simulink model "aes_impl_decrypt_smc"  (R2015b)
settings: Solver=FixedStepDiscrete  SolverMode=SingleTasking  StartTime=0.0  StopTime=1000e-6  RelTol=1e-3
undefined symbols (not defined in the file): a, b, input_sample_rate
libraries: shlslibv1 x3018
(part 11 of 20)

== system aes_impl_decrypt_smc/Round12/Subsystem8/Subsystem5/Mixcolumn1 ==
  In1 : Inport
  In2 : Inport  Port=2
  In3 : Inport  Port=3
  In4 : Inport  Port=4
  Binary Logic : shlslibv1/Math Functions/Binary Logic  syn_binlog_exp=a^b  synBlockType=primitive  synLatency=0  synBlockId=13
  Binary Logic1 : shlslibv1/Math Functions/Binary Logic  syn_binlog_exp=a^b  synBlockType=primitive  synLatency=0  synBlockId=13
  Binary Logic2 : shlslibv1/Math Functions/Binary Logic  syn_binlog_exp=a^b  synBlockType=primitive  synLatency=0  synBlockId=13
  Display5 : Display
      settings: Format=hex (Stored Integer)
  Port Out : shlslibv1/Ports & Subsystems/Port Out  syn_capture=on  syn_register=on  synBlockType=port  synLatency=1  synBlockId=1
  multiplier1 : shlslibv1/Memories/ROM  syn_rom_vec=mul11  syn_rom_auto_wl=on  syn_out_wl=8  syn_out_fl=0  syn_out_dt=unsigned  syn_out_sat=on  syn_out_rnd=on  syn_en_port=off  synBlockType=primitive  synLatency=1  synBlockId=62  syn_dual_port=off
  multiplier2 : shlslibv1/Memories/ROM  syn_rom_vec=mul9  syn_rom_auto_wl=on  syn_out_wl=8  syn_out_fl=0  syn_out_dt=unsigned  syn_out_sat=on  syn_out_rnd=on  syn_en_port=off  synBlockType=primitive  synLatency=1  synBlockId=62  syn_dual_port=off
  multiplier3 : shlslibv1/Memories/ROM  syn_rom_vec=mul14  syn_rom_auto_wl=on  syn_out_wl=8  syn_out_fl=0  syn_out_dt=unsigned  syn_out_sat=on  syn_out_rnd=on  syn_en_port=off  synBlockType=primitive  synLatency=1  synBlockId=62  syn_dual_port=off
  multiplier4 : shlslibv1/Memories/ROM  syn_rom_vec=mul13  syn_rom_auto_wl=on  syn_out_wl=8  syn_out_fl=0  syn_out_dt=unsigned  syn_out_sat=on  syn_out_rnd=on  syn_en_port=off  synBlockType=primitive  synLatency=1  synBlockId=62  syn_dual_port=off
  Out1 : Outport
  wires:
  multiplier3/1 -> Binary Logic/2
  In2/1 -> multiplier3/1
  multiplier2/1 -> Binary Logic/1
  Binary Logic2/1 -> Port Out/1, Out1/1
  In1/1 -> multiplier2/1
  Port Out/1 -> Display5/1
  Binary Logic/1 -> Binary Logic2/1
  Binary Logic1/1 -> Binary Logic2/2
  multiplier1/1 -> Binary Logic1/1
  In3/1 -> multiplier1/1
  multiplier4/1 -> Binary Logic1/2
  In4/1 -> multiplier4/1

== system aes_impl_decrypt_smc/Round12/Subsystem8/Subsystem5/Mixcolumn2 ==
  In1 : Inport
  In2 : Inport  Port=2
  In3 : Inport  Port=3
  In4 : Inport  Port=4
  Binary Logic : shlslibv1/Math Functions/Binary Logic  syn_binlog_exp=a^b  synBlockType=primitive  synLatency=0  synBlockId=13
  Binary Logic1 : shlslibv1/Math Functions/Binary Logic  syn_binlog_exp=a^b  synBlockType=primitive  synLatency=0  synBlockId=13
  Binary Logic2 : shlslibv1/Math Functions/Binary Logic  syn_binlog_exp=a^b  synBlockType=primitive  synLatency=0  synBlockId=13
  Display5 : Display
      settings: Format=hex (Stored Integer)
  Port Out : shlslibv1/Ports & Subsystems/Port Out  syn_capture=on  syn_register=on  synBlockType=port  synLatency=1  synBlockId=1
  multiplier1 : shlslibv1/Memories/ROM  syn_rom_vec=mul14  syn_rom_auto_wl=on  syn_out_wl=8  syn_out_fl=0  syn_out_dt=unsigned  syn_out_sat=on  syn_out_rnd=on  syn_en_port=off  synBlockType=primitive  synLatency=1  synBlockId=62  syn_dual_port=off
  multiplier2 : shlslibv1/Memories/ROM  syn_rom_vec=mul13  syn_rom_auto_wl=on  syn_out_wl=8  syn_out_fl=0  syn_out_dt=unsigned  syn_out_sat=on  syn_out_rnd=on  syn_en_port=off  synBlockType=primitive  synLatency=1  synBlockId=62  syn_dual_port=off
  multiplier3 : shlslibv1/Memories/ROM  syn_rom_vec=mul9  syn_rom_auto_wl=on  syn_out_wl=8  syn_out_fl=0  syn_out_dt=unsigned  syn_out_sat=on  syn_out_rnd=on  syn_en_port=off  synBlockType=primitive  synLatency=1  synBlockId=62  syn_dual_port=off
  multiplier4 : shlslibv1/Memories/ROM  syn_rom_vec=mul11  syn_rom_auto_wl=on  syn_out_wl=8  syn_out_fl=0  syn_out_dt=unsigned  syn_out_sat=on  syn_out_rnd=on  syn_en_port=off  synBlockType=primitive  synLatency=1  synBlockId=62  syn_dual_port=off
  Out1 : Outport
  wires:
  multiplier3/1 -> Binary Logic/2
  In2/1 -> multiplier3/1
  multiplier2/1 -> Binary Logic/1
  Binary Logic2/1 -> Port Out/1, Out1/1
  In1/1 -> multiplier2/1
  Port Out/1 -> Display5/1
  Binary Logic/1 -> Binary Logic2/1
  Binary Logic1/1 -> Binary Logic2/2
  multiplier1/1 -> Binary Logic1/1
  In3/1 -> multiplier1/1
  multiplier4/1 -> Binary Logic1/2
  In4/1 -> multiplier4/1

== system aes_impl_decrypt_smc/Round12/Subsystem8/Subsystem5/Mixcolumn3 ==
  In1 : Inport
  In2 : Inport  Port=2
  In3 : Inport  Port=3
  In4 : Inport  Port=4
  Binary Logic : shlslibv1/Math Functions/Binary Logic  syn_binlog_exp=a^b  synBlockType=primitive  synLatency=0  synBlockId=13
  Binary Logic1 : shlslibv1/Math Functions/Binary Logic  syn_binlog_exp=a^b  synBlockType=primitive  synLatency=0  synBlockId=13
  Binary Logic2 : shlslibv1/Math Functions/Binary Logic  syn_binlog_exp=a^b  synBlockType=primitive  synLatency=0  synBlockId=13
  Display5 : Display
      settings: Format=hex (Stored Integer)
  Port Out : shlslibv1/Ports & Subsystems/Port Out  syn_capture=on  syn_register=on  synBlockType=port  synLatency=1  synBlockId=1
  multiplier1 : shlslibv1/Memories/ROM  syn_rom_vec=mul9  syn_rom_auto_wl=on  syn_out_wl=8  syn_out_fl=0  syn_out_dt=unsigned  syn_out_sat=on  syn_out_rnd=on  syn_en_port=off  synBlockType=primitive  synLatency=1  synBlockId=62  syn_dual_port=off
  multiplier2 : shlslibv1/Memories/ROM  syn_rom_vec=mul11  syn_rom_auto_wl=on  syn_out_wl=8  syn_out_fl=0  syn_out_dt=unsigned  syn_out_sat=on  syn_out_rnd=on  syn_en_port=off  synBlockType=primitive  synLatency=1  synBlockId=62  syn_dual_port=off
  multiplier3 : shlslibv1/Memories/ROM  syn_rom_vec=mul13  syn_rom_auto_wl=on  syn_out_wl=8  syn_out_fl=0  syn_out_dt=unsigned  syn_out_sat=on  syn_out_rnd=on  syn_en_port=off  synBlockType=primitive  synLatency=1  synBlockId=62  syn_dual_port=off
  multiplier4 : shlslibv1/Memories/ROM  syn_rom_vec=mul14  syn_rom_auto_wl=on  syn_out_wl=8  syn_out_fl=0  syn_out_dt=unsigned  syn_out_sat=on  syn_out_rnd=on  syn_en_port=off  synBlockType=primitive  synLatency=1  synBlockId=62  syn_dual_port=off
  Out1 : Outport
  wires:
  multiplier3/1 -> Binary Logic/2
  In2/1 -> multiplier3/1
  multiplier2/1 -> Binary Logic/1
  Binary Logic2/1 -> Port Out/1, Out1/1
  In1/1 -> multiplier2/1
  Port Out/1 -> Display5/1
  Binary Logic/1 -> Binary Logic2/1
  Binary Logic1/1 -> Binary Logic2/2
  multiplier1/1 -> Binary Logic1/1
  In3/1 -> multiplier1/1
  multiplier4/1 -> Binary Logic1/2
  In4/1 -> multiplier4/1

== system aes_impl_decrypt_smc/Round12/Subsystem8/Subsystem6/Mixcolumn ==
  In1 : Inport
  In2 : Inport  Port=2
  In3 : Inport  Port=3
  In4 : Inport  Port=4
  Binary Logic : shlslibv1/Math Functions/Binary Logic  syn_binlog_exp=a^b  synBlockType=primitive  synLatency=0  synBlockId=13
  Binary Logic1 : shlslibv1/Math Functions/Binary Logic  syn_binlog_exp=a^b  synBlockType=primitive  synLatency=0  synBlockId=13
  Binary Logic2 : shlslibv1/Math Functions/Binary Logic  syn_binlog_exp=a^b  synBlockType=primitive  synLatency=0  synBlockId=13
  Display5 : Display
      settings: Format=hex (Stored Integer)
  Port Out : shlslibv1/Ports & Subsystems/Port Out  syn_capture=on  syn_register=on  synBlockType=port  synLatency=1  synBlockId=1
  multiplier1 : shlslibv1/Memories/ROM  syn_rom_vec=mul13  syn_rom_auto_wl=on  syn_out_wl=8  syn_out_fl=0  syn_out_dt=unsigned  syn_out_sat=on  syn_out_rnd=on  syn_en_port=off  synBlockType=primitive  synLatency=1  synBlockId=62  syn_dual_port=off
  multiplier2 : shlslibv1/Memories/ROM  syn_rom_vec=mul14  syn_rom_auto_wl=on  syn_out_wl=8  syn_out_fl=0  syn_out_dt=unsigned  syn_out_sat=on  syn_out_rnd=on  syn_en_port=off  synBlockType=primitive  synLatency=1  synBlockId=62  syn_dual_port=off
  multiplier3 : shlslibv1/Memories/ROM  syn_rom_vec=mul11  syn_rom_auto_wl=on  syn_out_wl=8  syn_out_fl=0  syn_out_dt=unsigned  syn_out_sat=on  syn_out_rnd=on  syn_en_port=off  synBlockType=primitive  synLatency=1  synBlockId=62  syn_dual_port=off
  multiplier4 : shlslibv1/Memories/ROM  syn_rom_vec=mul9  syn_rom_auto_wl=on  syn_out_wl=8  syn_out_fl=0  syn_out_dt=unsigned  syn_out_sat=on  syn_out_rnd=on  syn_en_port=off  synBlockType=primitive  synLatency=1  synBlockId=62  syn_dual_port=off
  Out1 : Outport
  wires:
  multiplier3/1 -> Binary Logic/2
  In2/1 -> multiplier3/1
  multiplier2/1 -> Binary Logic/1
  Binary Logic2/1 -> Port Out/1, Out1/1
  In1/1 -> multiplier2/1
  Port Out/1 -> Display5/1
  Binary Logic/1 -> Binary Logic2/1
  Binary Logic1/1 -> Binary Logic2/2
  multiplier1/1 -> Binary Logic1/1
  In3/1 -> multiplier1/1
  multiplier4/1 -> Binary Logic1/2
  In4/1 -> multiplier4/1

== system aes_impl_decrypt_smc/Round12/Subsystem8/Subsystem6/Mixcolumn1 ==
  In1 : Inport
  In2 : Inport  Port=2
  In3 : Inport  Port=3
  In4 : Inport  Port=4
  Binary Logic : shlslibv1/Math Functions/Binary Logic  syn_binlog_exp=a^b  synBlockType=primitive  synLatency=0  synBlockId=13
  Binary Logic1 : shlslibv1/Math Functions/Binary Logic  syn_binlog_exp=a^b  synBlockType=primitive  synLatency=0  synBlockId=13
  Binary Logic2 : shlslibv1/Math Functions/Binary Logic  syn_binlog_exp=a^b  synBlockType=primitive  synLatency=0  synBlockId=13
  Display5 : Display
      settings: Format=hex (Stored Integer)
  Port Out : shlslibv1/Ports & Subsystems/Port Out  syn_capture=on  syn_register=on  synBlockType=port  synLatency=1  synBlockId=1
  multiplier1 : shlslibv1/Memories/ROM  syn_rom_vec=mul11  syn_rom_auto_wl=on  syn_out_wl=8  syn_out_fl=0  syn_out_dt=unsigned  syn_out_sat=on  syn_out_rnd=on  syn_en_port=off  synBlockType=primitive  synLatency=1  synBlockId=62  syn_dual_port=off
  multiplier2 : shlslibv1/Memories/ROM  syn_rom_vec=mul9  syn_rom_auto_wl=on  syn_out_wl=8  syn_out_fl=0  syn_out_dt=unsigned  syn_out_sat=on  syn_out_rnd=on  syn_en_port=off  synBlockType=primitive  synLatency=1  synBlockId=62  syn_dual_port=off
  multiplier3 : shlslibv1/Memories/ROM  syn_rom_vec=mul14  syn_rom_auto_wl=on  syn_out_wl=8  syn_out_fl=0  syn_out_dt=unsigned  syn_out_sat=on  syn_out_rnd=on  syn_en_port=off  synBlockType=primitive  synLatency=1  synBlockId=62  syn_dual_port=off
  multiplier4 : shlslibv1/Memories/ROM  syn_rom_vec=mul13  syn_rom_auto_wl=on  syn_out_wl=8  syn_out_fl=0  syn_out_dt=unsigned  syn_out_sat=on  syn_out_rnd=on  syn_en_port=off  synBlockType=primitive  synLatency=1  synBlockId=62  syn_dual_port=off
  Out1 : Outport
  wires:
  multiplier3/1 -> Binary Logic/2
  In2/1 -> multiplier3/1
  multiplier2/1 -> Binary Logic/1
  Binary Logic2/1 -> Port Out/1, Out1/1
  In1/1 -> multiplier2/1
  Port Out/1 -> Display5/1
  Binary Logic/1 -> Binary Logic2/1
  Binary Logic1/1 -> Binary Logic2/2
  multiplier1/1 -> Binary Logic1/1
  In3/1 -> multiplier1/1
  multiplier4/1 -> Binary Logic1/2
  In4/1 -> multiplier4/1

== system aes_impl_decrypt_smc/Round12/Subsystem8/Subsystem6/Mixcolumn2 ==
  In1 : Inport
  In2 : Inport  Port=2
  In3 : Inport  Port=3
  In4 : Inport  Port=4
  Binary Logic : shlslibv1/Math Functions/Binary Logic  syn_binlog_exp=a^b  synBlockType=primitive  synLatency=0  synBlockId=13
  Binary Logic1 : shlslibv1/Math Functions/Binary Logic  syn_binlog_exp=a^b  synBlockType=primitive  synLatency=0  synBlockId=13
  Binary Logic2 : shlslibv1/Math Functions/Binary Logic  syn_binlog_exp=a^b  synBlockType=primitive  synLatency=0  synBlockId=13
  Display5 : Display
      settings: Format=hex (Stored Integer)
  Port Out : shlslibv1/Ports & Subsystems/Port Out  syn_capture=on  syn_register=on  synBlockType=port  synLatency=1  synBlockId=1
  multiplier1 : shlslibv1/Memories/ROM  syn_rom_vec=mul14  syn_rom_auto_wl=on  syn_out_wl=8  syn_out_fl=0  syn_out_dt=unsigned  syn_out_sat=on  syn_out_rnd=on  syn_en_port=off  synBlockType=primitive  synLatency=1  synBlockId=62  syn_dual_port=off
  multiplier2 : shlslibv1/Memories/ROM  syn_rom_vec=mul13  syn_rom_auto_wl=on  syn_out_wl=8  syn_out_fl=0  syn_out_dt=unsigned  syn_out_sat=on  syn_out_rnd=on  syn_en_port=off  synBlockType=primitive  synLatency=1  synBlockId=62  syn_dual_port=off
  multiplier3 : shlslibv1/Memories/ROM  syn_rom_vec=mul9  syn_rom_auto_wl=on  syn_out_wl=8  syn_out_fl=0  syn_out_dt=unsigned  syn_out_sat=on  syn_out_rnd=on  syn_en_port=off  synBlockType=primitive  synLatency=1  synBlockId=62  syn_dual_port=off
  multiplier4 : shlslibv1/Memories/ROM  syn_rom_vec=mul11  syn_rom_auto_wl=on  syn_out_wl=8  syn_out_fl=0  syn_out_dt=unsigned  syn_out_sat=on  syn_out_rnd=on  syn_en_port=off  synBlockType=primitive  synLatency=1  synBlockId=62  syn_dual_port=off
  Out1 : Outport
  wires:
  multiplier3/1 -> Binary Logic/2
  In2/1 -> multiplier3/1
  multiplier2/1 -> Binary Logic/1
  Binary Logic2/1 -> Port Out/1, Out1/1
  In1/1 -> multiplier2/1
  Port Out/1 -> Display5/1
  Binary Logic/1 -> Binary Logic2/1
  Binary Logic1/1 -> Binary Logic2/2
  multiplier1/1 -> Binary Logic1/1
  In3/1 -> multiplier1/1
  multiplier4/1 -> Binary Logic1/2
  In4/1 -> multiplier4/1

== system aes_impl_decrypt_smc/Round12/Subsystem8/Subsystem6/Mixcolumn3 ==
  In1 : Inport
  In2 : Inport  Port=2
  In3 : Inport  Port=3
  In4 : Inport  Port=4
  Binary Logic : shlslibv1/Math Functions/Binary Logic  syn_binlog_exp=a^b  synBlockType=primitive  synLatency=0  synBlockId=13
  Binary Logic1 : shlslibv1/Math Functions/Binary Logic  syn_binlog_exp=a^b  synBlockType=primitive  synLatency=0  synBlockId=13
  Binary Logic2 : shlslibv1/Math Functions/Binary Logic  syn_binlog_exp=a^b  synBlockType=primitive  synLatency=0  synBlockId=13
  Display5 : Display
      settings: Format=hex (Stored Integer)
  Port Out : shlslibv1/Ports & Subsystems/Port Out  syn_capture=on  syn_register=on  synBlockType=port  synLatency=1  synBlockId=1
  multiplier1 : shlslibv1/Memories/ROM  syn_rom_vec=mul9  syn_rom_auto_wl=on  syn_out_wl=8  syn_out_fl=0  syn_out_dt=unsigned  syn_out_sat=on  syn_out_rnd=on  syn_en_port=off  synBlockType=primitive  synLatency=1  synBlockId=62  syn_dual_port=off
  multiplier2 : shlslibv1/Memories/ROM  syn_rom_vec=mul11  syn_rom_auto_wl=on  syn_out_wl=8  syn_out_fl=0  syn_out_dt=unsigned  syn_out_sat=on  syn_out_rnd=on  syn_en_port=off  synBlockType=primitive  synLatency=1  synBlockId=62  syn_dual_port=off
  multiplier3 : shlslibv1/Memories/ROM  syn_rom_vec=mul13  syn_rom_auto_wl=on  syn_out_wl=8  syn_out_fl=0  syn_out_dt=unsigned  syn_out_sat=on  syn_out_rnd=on  syn_en_port=off  synBlockType=primitive  synLatency=1  synBlockId=62  syn_dual_port=off
  multiplier4 : shlslibv1/Memories/ROM  syn_rom_vec=mul14  syn_rom_auto_wl=on  syn_out_wl=8  syn_out_fl=0  syn_out_dt=unsigned  syn_out_sat=on  syn_out_rnd=on  syn_en_port=off  synBlockType=primitive  synLatency=1  synBlockId=62  syn_dual_port=off
  Out1 : Outport
  wires:
  multiplier3/1 -> Binary Logic/2
  In2/1 -> multiplier3/1
  multiplier2/1 -> Binary Logic/1
  Binary Logic2/1 -> Port Out/1, Out1/1
  In1/1 -> multiplier2/1
  Port Out/1 -> Display5/1
  Binary Logic/1 -> Binary Logic2/1
  Binary Logic1/1 -> Binary Logic2/2
  multiplier1/1 -> Binary Logic1/1
  In3/1 -> multiplier1/1
  multiplier4/1 -> Binary Logic1/2
  In4/1 -> multiplier4/1

== system aes_impl_decrypt_smc/Round12/Subsystem8/Subsystem7/Mixcolumn ==
  In1 : Inport
  In2 : Inport  Port=2
  In3 : Inport  Port=3
  In4 : Inport  Port=4
  Binary Logic : shlslibv1/Math Functions/Binary Logic  syn_binlog_exp=a^b  synBlockType=primitive  synLatency=0  synBlockId=13
  Binary Logic1 : shlslibv1/Math Functions/Binary Logic  syn_binlog_exp=a^b  synBlockType=primitive  synLatency=0  synBlockId=13
  Binary Logic2 : shlslibv1/Math Functions/Binary Logic  syn_binlog_exp=a^b  synBlockType=primitive  synLatency=0  synBlockId=13
  Display5 : Display
      settings: Format=hex (Stored Integer)
  Port Out : shlslibv1/Ports & Subsystems/Port Out  syn_capture=on  syn_register=on  synBlockType=port  synLatency=1  synBlockId=1
  multiplier1 : shlslibv1/Memories/ROM  syn_rom_vec=mul13  syn_rom_auto_wl=on  syn_out_wl=8  syn_out_fl=0  syn_out_dt=unsigned  syn_out_sat=on  syn_out_rnd=on  syn_en_port=off  synBlockType=primitive  synLatency=1  synBlockId=62  syn_dual_port=off
  multiplier2 : shlslibv1/Memories/ROM  syn_rom_vec=mul14  syn_rom_auto_wl=on  syn_out_wl=8  syn_out_fl=0  syn_out_dt=unsigned  syn_out_sat=on  syn_out_rnd=on  syn_en_port=off  synBlockType=primitive  synLatency=1  synBlockId=62  syn_dual_port=off
  multiplier3 : shlslibv1/Memories/ROM  syn_rom_vec=mul11  syn_rom_auto_wl=on  syn_out_wl=8  syn_out_fl=0  syn_out_dt=unsigned  syn_out_sat=on  syn_out_rnd=on  syn_en_port=off  synBlockType=primitive  synLatency=1  synBlockId=62  syn_dual_port=off
  multiplier4 : shlslibv1/Memories/ROM  syn_rom_vec=mul9  syn_rom_auto_wl=on  syn_out_wl=8  syn_out_fl=0  syn_out_dt=unsigned  syn_out_sat=on  syn_out_rnd=on  syn_en_port=off  synBlockType=primitive  synLatency=1  synBlockId=62  syn_dual_port=off
  Out1 : Outport
  wires:
  multiplier3/1 -> Binary Logic/2
  In2/1 -> multiplier3/1
  multiplier2/1 -> Binary Logic/1
  Binary Logic2/1 -> Port Out/1, Out1/1
  In1/1 -> multiplier2/1
  Port Out/1 -> Display5/1
  Binary Logic/1 -> Binary Logic2/1
  Binary Logic1/1 -> Binary Logic2/2
  multiplier1/1 -> Binary Logic1/1
  In3/1 -> multiplier1/1
  multiplier4/1 -> Binary Logic1/2
  In4/1 -> multiplier4/1

== system aes_impl_decrypt_smc/Round12/Subsystem8/Subsystem7/Mixcolumn1 ==
  In1 : Inport
  In2 : Inport  Port=2
  In3 : Inport  Port=3
  In4 : Inport  Port=4
  Binary Logic : shlslibv1/Math Functions/Binary Logic  syn_binlog_exp=a^b  synBlockType=primitive  synLatency=0  synBlockId=13
  Binary Logic1 : shlslibv1/Math Functions/Binary Logic  syn_binlog_exp=a^b  synBlockType=primitive  synLatency=0  synBlockId=13
  Binary Logic2 : shlslibv1/Math Functions/Binary Logic  syn_binlog_exp=a^b  synBlockType=primitive  synLatency=0  synBlockId=13
  Display5 : Display
      settings: Format=hex (Stored Integer)
  Port Out : shlslibv1/Ports & Subsystems/Port Out  syn_capture=on  syn_register=on  synBlockType=port  synLatency=1  synBlockId=1
  multiplier1 : shlslibv1/Memories/ROM  syn_rom_vec=mul11  syn_rom_auto_wl=on  syn_out_wl=8  syn_out_fl=0  syn_out_dt=unsigned  syn_out_sat=on  syn_out_rnd=on  syn_en_port=off  synBlockType=primitive  synLatency=1  synBlockId=62  syn_dual_port=off
  multiplier2 : shlslibv1/Memories/ROM  syn_rom_vec=mul9  syn_rom_auto_wl=on  syn_out_wl=8  syn_out_fl=0  syn_out_dt=unsigned  syn_out_sat=on  syn_out_rnd=on  syn_en_port=off  synBlockType=primitive  synLatency=1  synBlockId=62  syn_dual_port=off
  multiplier3 : shlslibv1/Memories/ROM  syn_rom_vec=mul14  syn_rom_auto_wl=on  syn_out_wl=8  syn_out_fl=0  syn_out_dt=unsigned  syn_out_sat=on  syn_out_rnd=on  syn_en_port=off  synBlockType=primitive  synLatency=1  synBlockId=62  syn_dual_port=off
  multiplier4 : shlslibv1/Memories/ROM  syn_rom_vec=mul13  syn_rom_auto_wl=on  syn_out_wl=8  syn_out_fl=0  syn_out_dt=unsigned  syn_out_sat=on  syn_out_rnd=on  syn_en_port=off  synBlockType=primitive  synLatency=1  synBlockId=62  syn_dual_port=off
  Out1 : Outport
  wires:
  multiplier3/1 -> Binary Logic/2
  In2/1 -> multiplier3/1
  multiplier2/1 -> Binary Logic/1
  Binary Logic2/1 -> Port Out/1, Out1/1
  In1/1 -> multiplier2/1
  Port Out/1 -> Display5/1
  Binary Logic/1 -> Binary Logic2/1
  Binary Logic1/1 -> Binary Logic2/2
  multiplier1/1 -> Binary Logic1/1
  In3/1 -> multiplier1/1
  multiplier4/1 -> Binary Logic1/2
  In4/1 -> multiplier4/1

== system aes_impl_decrypt_smc/Round12/Subsystem8/Subsystem7/Mixcolumn2 ==
  In1 : Inport
  In2 : Inport  Port=2
  In3 : Inport  Port=3
  In4 : Inport  Port=4
  Binary Logic : shlslibv1/Math Functions/Binary Logic  syn_binlog_exp=a^b  synBlockType=primitive  synLatency=0  synBlockId=13
  Binary Logic1 : shlslibv1/Math Functions/Binary Logic  syn_binlog_exp=a^b  synBlockType=primitive  synLatency=0  synBlockId=13
  Binary Logic2 : shlslibv1/Math Functions/Binary Logic  syn_binlog_exp=a^b  synBlockType=primitive  synLatency=0  synBlockId=13
  Display5 : Display
      settings: Format=hex (Stored Integer)
  Port Out : shlslibv1/Ports & Subsystems/Port Out  syn_capture=on  syn_register=on  synBlockType=port  synLatency=1  synBlockId=1
  multiplier1 : shlslibv1/Memories/ROM  syn_rom_vec=mul14  syn_rom_auto_wl=on  syn_out_wl=8  syn_out_fl=0  syn_out_dt=unsigned  syn_out_sat=on  syn_out_rnd=on  syn_en_port=off  synBlockType=primitive  synLatency=1  synBlockId=62  syn_dual_port=off
  multiplier2 : shlslibv1/Memories/ROM  syn_rom_vec=mul13  syn_rom_auto_wl=on  syn_out_wl=8  syn_out_fl=0  syn_out_dt=unsigned  syn_out_sat=on  syn_out_rnd=on  syn_en_port=off  synBlockType=primitive  synLatency=1  synBlockId=62  syn_dual_port=off
  multiplier3 : shlslibv1/Memories/ROM  syn_rom_vec=mul9  syn_rom_auto_wl=on  syn_out_wl=8  syn_out_fl=0  syn_out_dt=unsigned  syn_out_sat=on  syn_out_rnd=on  syn_en_port=off  synBlockType=primitive  synLatency=1  synBlockId=62  syn_dual_port=off
  multiplier4 : shlslibv1/Memories/ROM  syn_rom_vec=mul11  syn_rom_auto_wl=on  syn_out_wl=8  syn_out_fl=0  syn_out_dt=unsigned  syn_out_sat=on  syn_out_rnd=on  syn_en_port=off  synBlockType=primitive  synLatency=1  synBlockId=62  syn_dual_port=off
  Out1 : Outport
  wires:
  multiplier3/1 -> Binary Logic/2
  In2/1 -> multiplier3/1
  multiplier2/1 -> Binary Logic/1
  Binary Logic2/1 -> Port Out/1, Out1/1
  In1/1 -> multiplier2/1
  Port Out/1 -> Display5/1
  Binary Logic/1 -> Binary Logic2/1
  Binary Logic1/1 -> Binary Logic2/2
  multiplier1/1 -> Binary Logic1/1
  In3/1 -> multiplier1/1
  multiplier4/1 -> Binary Logic1/2
  In4/1 -> multiplier4/1

== system aes_impl_decrypt_smc/Round12/Subsystem8/Subsystem7/Mixcolumn3 ==
  In1 : Inport
  In2 : Inport  Port=2
  In3 : Inport  Port=3
  In4 : Inport  Port=4
  Binary Logic : shlslibv1/Math Functions/Binary Logic  syn_binlog_exp=a^b  synBlockType=primitive  synLatency=0  synBlockId=13
  Binary Logic1 : shlslibv1/Math Functions/Binary Logic  syn_binlog_exp=a^b  synBlockType=primitive  synLatency=0  synBlockId=13
  Binary Logic2 : shlslibv1/Math Functions/Binary Logic  syn_binlog_exp=a^b  synBlockType=primitive  synLatency=0  synBlockId=13
  Display5 : Display
      settings: Format=hex (Stored Integer)
  Port Out : shlslibv1/Ports & Subsystems/Port Out  syn_capture=on  syn_register=on  synBlockType=port  synLatency=1  synBlockId=1
  multiplier1 : shlslibv1/Memories/ROM  syn_rom_vec=mul9  syn_rom_auto_wl=on  syn_out_wl=8  syn_out_fl=0  syn_out_dt=unsigned  syn_out_sat=on  syn_out_rnd=on  syn_en_port=off  synBlockType=primitive  synLatency=1  synBlockId=62  syn_dual_port=off
  multiplier2 : shlslibv1/Memories/ROM  syn_rom_vec=mul11  syn_rom_auto_wl=on  syn_out_wl=8  syn_out_fl=0  syn_out_dt=unsigned  syn_out_sat=on  syn_out_rnd=on  syn_en_port=off  synBlockType=primitive  synLatency=1  synBlockId=62  syn_dual_port=off
  multiplier3 : shlslibv1/Memories/ROM  syn_rom_vec=mul13  syn_rom_auto_wl=on  syn_out_wl=8  syn_out_fl=0  syn_out_dt=unsigned  syn_out_sat=on  syn_out_rnd=on  syn_en_port=off  synBlockType=primitive  synLatency=1  synBlockId=62  syn_dual_port=off
  multiplier4 : shlslibv1/Memories/ROM  syn_rom_vec=mul14  syn_rom_auto_wl=on  syn_out_wl=8  syn_out_fl=0  syn_out_dt=unsigned  syn_out_sat=on  syn_out_rnd=on  syn_en_port=off  synBlockType=primitive  synLatency=1  synBlockId=62  syn_dual_port=off
  Out1 : Outport
  wires:
  multiplier3/1 -> Binary Logic/2
  In2/1 -> multiplier3/1
  multiplier2/1 -> Binary Logic/1
  Binary Logic2/1 -> Port Out/1, Out1/1
  In1/1 -> multiplier2/1
  Port Out/1 -> Display5/1
  Binary Logic/1 -> Binary Logic2/1
  Binary Logic1/1 -> Binary Logic2/2
  multiplier1/1 -> Binary Logic1/1
  In3/1 -> multiplier1/1
  multiplier4/1 -> Binary Logic1/2
  In4/1 -> multiplier4/1

== system aes_impl_decrypt_smc/Round12/Subsystem8/Subsystem8/Mixcolumn ==
  In1 : Inport
  In2 : Inport  Port=2
  In3 : Inport  Port=3
  In4 : Inport  Port=4
  Binary Logic : shlslibv1/Math Functions/Binary Logic  syn_binlog_exp=a^b  synBlockType=primitive  synLatency=0  synBlockId=13
  Binary Logic1 : shlslibv1/Math Functions/Binary Logic  syn_binlog_exp=a^b  synBlockType=primitive  synLatency=0  synBlockId=13
  Binary Logic2 : shlslibv1/Math Functions/Binary Logic  syn_binlog_exp=a^b  synBlockType=primitive  synLatency=0  synBlockId=13
  Display5 : Display
      settings: Format=hex (Stored Integer)
  Port Out : shlslibv1/Ports & Subsystems/Port Out  syn_capture=on  syn_register=on  synBlockType=port  synLatency=1  synBlockId=1
  multiplier1 : shlslibv1/Memories/ROM  syn_rom_vec=mul13  syn_rom_auto_wl=on  syn_out_wl=8  syn_out_fl=0  syn_out_dt=unsigned  syn_out_sat=on  syn_out_rnd=on  syn_en_port=off  synBlockType=primitive  synLatency=1  synBlockId=62  syn_dual_port=off
  multiplier2 : shlslibv1/Memories/ROM  syn_rom_vec=mul14  syn_rom_auto_wl=on  syn_out_wl=8  syn_out_fl=0  syn_out_dt=unsigned  syn_out_sat=on  syn_out_rnd=on  syn_en_port=off  synBlockType=primitive  synLatency=1  synBlockId=62  syn_dual_port=off
  multiplier3 : shlslibv1/Memories/ROM  syn_rom_vec=mul11  syn_rom_auto_wl=on  syn_out_wl=8  syn_out_fl=0  syn_out_dt=unsigned  syn_out_sat=on  syn_out_rnd=on  syn_en_port=off  synBlockType=primitive  synLatency=1  synBlockId=62  syn_dual_port=off
  multiplier4 : shlslibv1/Memories/ROM  syn_rom_vec=mul9  syn_rom_auto_wl=on  syn_out_wl=8  syn_out_fl=0  syn_out_dt=unsigned  syn_out_sat=on  syn_out_rnd=on  syn_en_port=off  synBlockType=primitive  synLatency=1  synBlockId=62  syn_dual_port=off
  Out1 : Outport
  wires:
  multiplier3/1 -> Binary Logic/2
  In2/1 -> multiplier3/1
  multiplier2/1 -> Binary Logic/1
  Binary Logic2/1 -> Port Out/1, Out1/1
  In1/1 -> multiplier2/1
  Port Out/1 -> Display5/1
  Binary Logic/1 -> Binary Logic2/1
  Binary Logic1/1 -> Binary Logic2/2
  multiplier1/1 -> Binary Logic1/1
  In3/1 -> multiplier1/1
  multiplier4/1 -> Binary Logic1/2
  In4/1 -> multiplier4/1

== system aes_impl_decrypt_smc/Round12/Subsystem8/Subsystem8/Mixcolumn1 ==
  In1 : Inport
  In2 : Inport  Port=2
  In3 : Inport  Port=3
  In4 : Inport  Port=4
  Binary Logic : shlslibv1/Math Functions/Binary Logic  syn_binlog_exp=a^b  synBlockType=primitive  synLatency=0  synBlockId=13
  Binary Logic1 : shlslibv1/Math Functions/Binary Logic  syn_binlog_exp=a^b  synBlockType=primitive  synLatency=0  synBlockId=13
  Binary Logic2 : shlslibv1/Math Functions/Binary Logic  syn_binlog_exp=a^b  synBlockType=primitive  synLatency=0  synBlockId=13
  Display5 : Display
      settings: Format=hex (Stored Integer)
  Port Out : shlslibv1/Ports & Subsystems/Port Out  syn_capture=on  syn_register=on  synBlockType=port  synLatency=1  synBlockId=1
  multiplier1 : shlslibv1/Memories/ROM  syn_rom_vec=mul11  syn_rom_auto_wl=on  syn_out_wl=8  syn_out_fl=0  syn_out_dt=unsigned  syn_out_sat=on  syn_out_rnd=on  syn_en_port=off  synBlockType=primitive  synLatency=1  synBlockId=62  syn_dual_port=off
  multiplier2 : shlslibv1/Memories/ROM  syn_rom_vec=mul9  syn_rom_auto_wl=on  syn_out_wl=8  syn_out_fl=0  syn_out_dt=unsigned  syn_out_sat=on  syn_out_rnd=on  syn_en_port=off  synBlockType=primitive  synLatency=1  synBlockId=62  syn_dual_port=off
  multiplier3 : shlslibv1/Memories/ROM  syn_rom_vec=mul14  syn_rom_auto_wl=on  syn_out_wl=8  syn_out_fl=0  syn_out_dt=unsigned  syn_out_sat=on  syn_out_rnd=on  syn_en_port=off  synBlockType=primitive  synLatency=1  synBlockId=62  syn_dual_port=off
  multiplier4 : shlslibv1/Memories/ROM  syn_rom_vec=mul13  syn_rom_auto_wl=on  syn_out_wl=8  syn_out_fl=0  syn_out_dt=unsigned  syn_out_sat=on  syn_out_rnd=on  syn_en_port=off  synBlockType=primitive  synLatency=1  synBlockId=62  syn_dual_port=off
  Out1 : Outport
  wires:
  multiplier3/1 -> Binary Logic/2
  In2/1 -> multiplier3/1
  multiplier2/1 -> Binary Logic/1
  Binary Logic2/1 -> Port Out/1, Out1/1
  In1/1 -> multiplier2/1
  Port Out/1 -> Display5/1
  Binary Logic/1 -> Binary Logic2/1
  Binary Logic1/1 -> Binary Logic2/2
  multiplier1/1 -> Binary Logic1/1
  In3/1 -> multiplier1/1
  multiplier4/1 -> Binary Logic1/2
  In4/1 -> multiplier4/1

== system aes_impl_decrypt_smc/Round12/Subsystem8/Subsystem8/Mixcolumn2 ==
  In1 : Inport
  In2 : Inport  Port=2
  In3 : Inport  Port=3
  In4 : Inport  Port=4
  Binary Logic : shlslibv1/Math Functions/Binary Logic  syn_binlog_exp=a^b  synBlockType=primitive  synLatency=0  synBlockId=13
  Binary Logic1 : shlslibv1/Math Functions/Binary Logic  syn_binlog_exp=a^b  synBlockType=primitive  synLatency=0  synBlockId=13
  Binary Logic2 : shlslibv1/Math Functions/Binary Logic  syn_binlog_exp=a^b  synBlockType=primitive  synLatency=0  synBlockId=13
  Display5 : Display
      settings: Format=hex (Stored Integer)
  Port Out : shlslibv1/Ports & Subsystems/Port Out  syn_capture=on  syn_register=on  synBlockType=port  synLatency=1  synBlockId=1
  multiplier1 : shlslibv1/Memories/ROM  syn_rom_vec=mul14  syn_rom_auto_wl=on  syn_out_wl=8  syn_out_fl=0  syn_out_dt=unsigned  syn_out_sat=on  syn_out_rnd=on  syn_en_port=off  synBlockType=primitive  synLatency=1  synBlockId=62  syn_dual_port=off
  multiplier2 : shlslibv1/Memories/ROM  syn_rom_vec=mul13  syn_rom_auto_wl=on  syn_out_wl=8  syn_out_fl=0  syn_out_dt=unsigned  syn_out_sat=on  syn_out_rnd=on  syn_en_port=off  synBlockType=primitive  synLatency=1  synBlockId=62  syn_dual_port=off
  multiplier3 : shlslibv1/Memories/ROM  syn_rom_vec=mul9  syn_rom_auto_wl=on  syn_out_wl=8  syn_out_fl=0  syn_out_dt=unsigned  syn_out_sat=on  syn_out_rnd=on  syn_en_port=off  synBlockType=primitive  synLatency=1  synBlockId=62  syn_dual_port=off
  multiplier4 : shlslibv1/Memories/ROM  syn_rom_vec=mul11  syn_rom_auto_wl=on  syn_out_wl=8  syn_out_fl=0  syn_out_dt=unsigned  syn_out_sat=on  syn_out_rnd=on  syn_en_port=off  synBlockType=primitive  synLatency=1  synBlockId=62  syn_dual_port=off
  Out1 : Outport
  wires:
  multiplier3/1 -> Binary Logic/2
  In2/1 -> multiplier3/1
  multiplier2/1 -> Binary Logic/1
  Binary Logic2/1 -> Port Out/1, Out1/1
  In1/1 -> multiplier2/1
  Port Out/1 -> Display5/1
  Binary Logic/1 -> Binary Logic2/1
  Binary Logic1/1 -> Binary Logic2/2
  multiplier1/1 -> Binary Logic1/1
  In3/1 -> multiplier1/1
  multiplier4/1 -> Binary Logic1/2
  In4/1 -> multiplier4/1

== system aes_impl_decrypt_smc/Round12/Subsystem8/Subsystem8/Mixcolumn3 ==
  In1 : Inport
  In2 : Inport  Port=2
  In3 : Inport  Port=3
  In4 : Inport  Port=4
  Binary Logic : shlslibv1/Math Functions/Binary Logic  syn_binlog_exp=a^b  synBlockType=primitive  synLatency=0  synBlockId=13
  Binary Logic1 : shlslibv1/Math Functions/Binary Logic  syn_binlog_exp=a^b  synBlockType=primitive  synLatency=0  synBlockId=13
  Binary Logic2 : shlslibv1/Math Functions/Binary Logic  syn_binlog_exp=a^b  synBlockType=primitive  synLatency=0  synBlockId=13
  Display5 : Display
      settings: Format=hex (Stored Integer)
  Port Out : shlslibv1/Ports & Subsystems/Port Out  syn_capture=on  syn_register=on  synBlockType=port  synLatency=1  synBlockId=1
  multiplier1 : shlslibv1/Memories/ROM  syn_rom_vec=mul9  syn_rom_auto_wl=on  syn_out_wl=8  syn_out_fl=0  syn_out_dt=unsigned  syn_out_sat=on  syn_out_rnd=on  syn_en_port=off  synBlockType=primitive  synLatency=1  synBlockId=62  syn_dual_port=off
  multiplier2 : shlslibv1/Memories/ROM  syn_rom_vec=mul11  syn_rom_auto_wl=on  syn_out_wl=8  syn_out_fl=0  syn_out_dt=unsigned  syn_out_sat=on  syn_out_rnd=on  syn_en_port=off  synBlockType=primitive  synLatency=1  synBlockId=62  syn_dual_port=off
  multiplier3 : shlslibv1/Memories/ROM  syn_rom_vec=mul13  syn_rom_auto_wl=on  syn_out_wl=8  syn_out_fl=0  syn_out_dt=unsigned  syn_out_sat=on  syn_out_rnd=on  syn_en_port=off  synBlockType=primitive  synLatency=1  synBlockId=62  syn_dual_port=off
  multiplier4 : shlslibv1/Memories/ROM  syn_rom_vec=mul14  syn_rom_auto_wl=on  syn_out_wl=8  syn_out_fl=0  syn_out_dt=unsigned  syn_out_sat=on  syn_out_rnd=on  syn_en_port=off  synBlockType=primitive  synLatency=1  synBlockId=62  syn_dual_port=off
  Out1 : Outport
  wires:
  multiplier3/1 -> Binary Logic/2
  In2/1 -> multiplier3/1
  multiplier2/1 -> Binary Logic/1
  Binary Logic2/1 -> Port Out/1, Out1/1
  In1/1 -> multiplier2/1
  Port Out/1 -> Display5/1
  Binary Logic/1 -> Binary Logic2/1
  Binary Logic1/1 -> Binary Logic2/2
  multiplier1/1 -> Binary Logic1/1
  In3/1 -> multiplier1/1
  multiplier4/1 -> Binary Logic1/2
  In4/1 -> multiplier4/1

== system aes_impl_decrypt_smc/Round14/Subsystem8/Subsystem5/Mixcolumn ==
  In1 : Inport
  In2 : Inport  Port=2
  In3 : Inport  Port=3
  In4 : Inport  Port=4
  Binary Logic : shlslibv1/Math Functions/Binary Logic  syn_binlog_exp=a^b  synBlockType=primitive  synLatency=0  synBlockId=13
  Binary Logic1 : shlslibv1/Math Functions/Binary Logic  syn_binlog_exp=a^b  synBlockType=primitive  synLatency=0  synBlockId=13
  Binary Logic2 : shlslibv1/Math Functions/Binary Logic  syn_binlog_exp=a^b  synBlockType=primitive  synLatency=0  synBlockId=13
  Display5 : Display
      settings: Format=hex (Stored Integer)
  Port Out : shlslibv1/Ports & Subsystems/Port Out  syn_capture=on  syn_register=on  synBlockType=port  synLatency=1  synBlockId=1
  multiplier1 : shlslibv1/Memories/ROM  syn_rom_vec=mul13  syn_rom_auto_wl=on  syn_out_wl=8  syn_out_fl=0  syn_out_dt=unsigned  syn_out_sat=on  syn_out_rnd=on  syn_en_port=off  synBlockType=primitive  synLatency=1  synBlockId=62  syn_dual_port=off
  multiplier2 : shlslibv1/Memories/ROM  syn_rom_vec=mul14  syn_rom_auto_wl=on  syn_out_wl=8  syn_out_fl=0  syn_out_dt=unsigned  syn_out_sat=on  syn_out_rnd=on  syn_en_port=off  synBlockType=primitive  synLatency=1  synBlockId=62  syn_dual_port=off
  multiplier3 : shlslibv1/Memories/ROM  syn_rom_vec=mul11  syn_rom_auto_wl=on  syn_out_wl=8  syn_out_fl=0  syn_out_dt=unsigned  syn_out_sat=on  syn_out_rnd=on  syn_en_port=off  synBlockType=primitive  synLatency=1  synBlockId=62  syn_dual_port=off
  multiplier4 : shlslibv1/Memories/ROM  syn_rom_vec=mul9  syn_rom_auto_wl=on  syn_out_wl=8  syn_out_fl=0  syn_out_dt=unsigned  syn_out_sat=on  syn_out_rnd=on  syn_en_port=off  synBlockType=primitive  synLatency=1  synBlockId=62  syn_dual_port=off
  Out1 : Outport
  wires:
  multiplier3/1 -> Binary Logic/2
  In2/1 -> multiplier3/1
  multiplier2/1 -> Binary Logic/1
  Binary Logic2/1 -> Port Out/1, Out1/1
  In1/1 -> multiplier2/1
  Port Out/1 -> Display5/1
  Binary Logic/1 -> Binary Logic2/1
  Binary Logic1/1 -> Binary Logic2/2
  multiplier1/1 -> Binary Logic1/1
  In3/1 -> multiplier1/1
  multiplier4/1 -> Binary Logic1/2
  In4/1 -> multiplier4/1

== system aes_impl_decrypt_smc/Round14/Subsystem8/Subsystem5/Mixcolumn1 ==
  In1 : Inport
  In2 : Inport  Port=2
  In3 : Inport  Port=3
  In4 : Inport  Port=4
  Binary Logic : shlslibv1/Math Functions/Binary Logic  syn_binlog_exp=a^b  synBlockType=primitive  synLatency=0  synBlockId=13
  Binary Logic1 : shlslibv1/Math Functions/Binary Logic  syn_binlog_exp=a^b  synBlockType=primitive  synLatency=0  synBlockId=13
  Binary Logic2 : shlslibv1/Math Functions/Binary Logic  syn_binlog_exp=a^b  synBlockType=primitive  synLatency=0  synBlockId=13
  Display5 : Display
      settings: Format=hex (Stored Integer)
  Port Out : shlslibv1/Ports & Subsystems/Port Out  syn_capture=on  syn_register=on  synBlockType=port  synLatency=1  synBlockId=1
  multiplier1 : shlslibv1/Memories/ROM  syn_rom_vec=mul11  syn_rom_auto_wl=on  syn_out_wl=8  syn_out_fl=0  syn_out_dt=unsigned  syn_out_sat=on  syn_out_rnd=on  syn_en_port=off  synBlockType=primitive  synLatency=1  synBlockId=62  syn_dual_port=off
  multiplier2 : shlslibv1/Memories/ROM  syn_rom_vec=mul9  syn_rom_auto_wl=on  syn_out_wl=8  syn_out_fl=0  syn_out_dt=unsigned  syn_out_sat=on  syn_out_rnd=on  syn_en_port=off  synBlockType=primitive  synLatency=1  synBlockId=62  syn_dual_port=off
  multiplier3 : shlslibv1/Memories/ROM  syn_rom_vec=mul14  syn_rom_auto_wl=on  syn_out_wl=8  syn_out_fl=0  syn_out_dt=unsigned  syn_out_sat=on  syn_out_rnd=on  syn_en_port=off  synBlockType=primitive  synLatency=1  synBlockId=62  syn_dual_port=off
  multiplier4 : shlslibv1/Memories/ROM  syn_rom_vec=mul13  syn_rom_auto_wl=on  syn_out_wl=8  syn_out_fl=0  syn_out_dt=unsigned  syn_out_sat=on  syn_out_rnd=on  syn_en_port=off  synBlockType=primitive  synLatency=1  synBlockId=62  syn_dual_port=off
  Out1 : Outport
  wires:
  multiplier3/1 -> Binary Logic/2
  In2/1 -> multiplier3/1
  multiplier2/1 -> Binary Logic/1
  Binary Logic2/1 -> Port Out/1, Out1/1
  In1/1 -> multiplier2/1
  Port Out/1 -> Display5/1
  Binary Logic/1 -> Binary Logic2/1
  Binary Logic1/1 -> Binary Logic2/2
  multiplier1/1 -> Binary Logic1/1
  In3/1 -> multiplier1/1
  multiplier4/1 -> Binary Logic1/2
  In4/1 -> multiplier4/1

== system aes_impl_decrypt_smc/Round14/Subsystem8/Subsystem5/Mixcolumn2 ==
  In1 : Inport
  In2 : Inport  Port=2
  In3 : Inport  Port=3
  In4 : Inport  Port=4
  Binary Logic : shlslibv1/Math Functions/Binary Logic  syn_binlog_exp=a^b  synBlockType=primitive  synLatency=0  synBlockId=13
  Binary Logic1 : shlslibv1/Math Functions/Binary Logic  syn_binlog_exp=a^b  synBlockType=primitive  synLatency=0  synBlockId=13
  Binary Logic2 : shlslibv1/Math Functions/Binary Logic  syn_binlog_exp=a^b  synBlockType=primitive  synLatency=0  synBlockId=13
  Display5 : Display
      settings: Format=hex (Stored Integer)
  Port Out : shlslibv1/Ports & Subsystems/Port Out  syn_capture=on  syn_register=on  synBlockType=port  synLatency=1  synBlockId=1
  multiplier1 : shlslibv1/Memories/ROM  syn_rom_vec=mul14  syn_rom_auto_wl=on  syn_out_wl=8  syn_out_fl=0  syn_out_dt=unsigned  syn_out_sat=on  syn_out_rnd=on  syn_en_port=off  synBlockType=primitive  synLatency=1  synBlockId=62  syn_dual_port=off
  multiplier2 : shlslibv1/Memories/ROM  syn_rom_vec=mul13  syn_rom_auto_wl=on  syn_out_wl=8  syn_out_fl=0  syn_out_dt=unsigned  syn_out_sat=on  syn_out_rnd=on  syn_en_port=off  synBlockType=primitive  synLatency=1  synBlockId=62  syn_dual_port=off
  multiplier3 : shlslibv1/Memories/ROM  syn_rom_vec=mul9  syn_rom_auto_wl=on  syn_out_wl=8  syn_out_fl=0  syn_out_dt=unsigned  syn_out_sat=on  syn_out_rnd=on  syn_en_port=off  synBlockType=primitive  synLatency=1  synBlockId=62  syn_dual_port=off
  multiplier4 : shlslibv1/Memories/ROM  syn_rom_vec=mul11  syn_rom_auto_wl=on  syn_out_wl=8  syn_out_fl=0  syn_out_dt=unsigned  syn_out_sat=on  syn_out_rnd=on  syn_en_port=off  synBlockType=primitive  synLatency=1  synBlockId=62  syn_dual_port=off
  Out1 : Outport
  wires:
  multiplier3/1 -> Binary Logic/2
  In2/1 -> multiplier3/1
  multiplier2/1 -> Binary Logic/1
  Binary Logic2/1 -> Port Out/1, Out1/1
  In1/1 -> multiplier2/1
  Port Out/1 -> Display5/1
  Binary Logic/1 -> Binary Logic2/1
  Binary Logic1/1 -> Binary Logic2/2
  multiplier1/1 -> Binary Logic1/1
  In3/1 -> multiplier1/1
  multiplier4/1 -> Binary Logic1/2
  In4/1 -> multiplier4/1

== system aes_impl_decrypt_smc/Round14/Subsystem8/Subsystem5/Mixcolumn3 ==
  In1 : Inport
  In2 : Inport  Port=2
  In3 : Inport  Port=3
  In4 : Inport  Port=4
  Binary Logic : shlslibv1/Math Functions/Binary Logic  syn_binlog_exp=a^b  synBlockType=primitive  synLatency=0  synBlockId=13
  Binary Logic1 : shlslibv1/Math Functions/Binary Logic  syn_binlog_exp=a^b  synBlockType=primitive  synLatency=0  synBlockId=13
  Binary Logic2 : shlslibv1/Math Functions/Binary Logic  syn_binlog_exp=a^b  synBlockType=primitive  synLatency=0  synBlockId=13
  Display5 : Display
      settings: Format=hex (Stored Integer)
  Port Out : shlslibv1/Ports & Subsystems/Port Out  syn_capture=on  syn_register=on  synBlockType=port  synLatency=1  synBlockId=1
  multiplier1 : shlslibv1/Memories/ROM  syn_rom_vec=mul9  syn_rom_auto_wl=on  syn_out_wl=8  syn_out_fl=0  syn_out_dt=unsigned  syn_out_sat=on  syn_out_rnd=on  syn_en_port=off  synBlockType=primitive  synLatency=1  synBlockId=62  syn_dual_port=off
  multiplier2 : shlslibv1/Memories/ROM  syn_rom_vec=mul11  syn_rom_auto_wl=on  syn_out_wl=8  syn_out_fl=0  syn_out_dt=unsigned  syn_out_sat=on  syn_out_rnd=on  syn_en_port=off  synBlockType=primitive  synLatency=1  synBlockId=62  syn_dual_port=off
  multiplier3 : shlslibv1/Memories/ROM  syn_rom_vec=mul13  syn_rom_auto_wl=on  syn_out_wl=8  syn_out_fl=0  syn_out_dt=unsigned  syn_out_sat=on  syn_out_rnd=on  syn_en_port=off  synBlockType=primitive  synLatency=1  synBlockId=62  syn_dual_port=off
  multiplier4 : shlslibv1/Memories/ROM  syn_rom_vec=mul14  syn_rom_auto_wl=on  syn_out_wl=8  syn_out_fl=0  syn_out_dt=unsigned  syn_out_sat=on  syn_out_rnd=on  syn_en_port=off  synBlockType=primitive  synLatency=1  synBlockId=62  syn_dual_port=off
  Out1 : Outport
  wires:
  multiplier3/1 -> Binary Logic/2
  In2/1 -> multiplier3/1
  multiplier2/1 -> Binary Logic/1
  Binary Logic2/1 -> Port Out/1, Out1/1
  In1/1 -> multiplier2/1
  Port Out/1 -> Display5/1
  Binary Logic/1 -> Binary Logic2/1
  Binary Logic1/1 -> Binary Logic2/2
  multiplier1/1 -> Binary Logic1/1
  In3/1 -> multiplier1/1
  multiplier4/1 -> Binary Logic1/2
  In4/1 -> multiplier4/1

== system aes_impl_decrypt_smc/Round14/Subsystem8/Subsystem6/Mixcolumn ==
  In1 : Inport
  In2 : Inport  Port=2
  In3 : Inport  Port=3
  In4 : Inport  Port=4
  Binary Logic : shlslibv1/Math Functions/Binary Logic  syn_binlog_exp=a^b  synBlockType=primitive  synLatency=0  synBlockId=13
  Binary Logic1 : shlslibv1/Math Functions/Binary Logic  syn_binlog_exp=a^b  synBlockType=primitive  synLatency=0  synBlockId=13
  Binary Logic2 : shlslibv1/Math Functions/Binary Logic  syn_binlog_exp=a^b  synBlockType=primitive  synLatency=0  synBlockId=13
  Display5 : Display
      settings: Format=hex (Stored Integer)
  Port Out : shlslibv1/Ports & Subsystems/Port Out  syn_capture=on  syn_register=on  synBlockType=port  synLatency=1  synBlockId=1
  multiplier1 : shlslibv1/Memories/ROM  syn_rom_vec=mul13  syn_rom_auto_wl=on  syn_out_wl=8  syn_out_fl=0  syn_out_dt=unsigned  syn_out_sat=on  syn_out_rnd=on  syn_en_port=off  synBlockType=primitive  synLatency=1  synBlockId=62  syn_dual_port=off
  multiplier2 : shlslibv1/Memories/ROM  syn_rom_vec=mul14  syn_rom_auto_wl=on  syn_out_wl=8  syn_out_fl=0  syn_out_dt=unsigned  syn_out_sat=on  syn_out_rnd=on  syn_en_port=off  synBlockType=primitive  synLatency=1  synBlockId=62  syn_dual_port=off
  multiplier3 : shlslibv1/Memories/ROM  syn_rom_vec=mul11  syn_rom_auto_wl=on  syn_out_wl=8  syn_out_fl=0  syn_out_dt=unsigned  syn_out_sat=on  syn_out_rnd=on  syn_en_port=off  synBlockType=primitive  synLatency=1  synBlockId=62  syn_dual_port=off
  multiplier4 : shlslibv1/Memories/ROM  syn_rom_vec=mul9  syn_rom_auto_wl=on  syn_out_wl=8  syn_out_fl=0  syn_out_dt=unsigned  syn_out_sat=on  syn_out_rnd=on  syn_en_port=off  synBlockType=primitive  synLatency=1  synBlockId=62  syn_dual_port=off
  Out1 : Outport
  wires:
  multiplier3/1 -> Binary Logic/2
  In2/1 -> multiplier3/1
  multiplier2/1 -> Binary Logic/1
  Binary Logic2/1 -> Port Out/1, Out1/1
  In1/1 -> multiplier2/1
  Port Out/1 -> Display5/1
  Binary Logic/1 -> Binary Logic2/1
  Binary Logic1/1 -> Binary Logic2/2
  multiplier1/1 -> Binary Logic1/1
  In3/1 -> multiplier1/1
  multiplier4/1 -> Binary Logic1/2
  In4/1 -> multiplier4/1

== system aes_impl_decrypt_smc/Round14/Subsystem8/Subsystem6/Mixcolumn1 ==
  In1 : Inport
  In2 : Inport  Port=2
  In3 : Inport  Port=3
  In4 : Inport  Port=4
  Binary Logic : shlslibv1/Math Functions/Binary Logic  syn_binlog_exp=a^b  synBlockType=primitive  synLatency=0  synBlockId=13
  Binary Logic1 : shlslibv1/Math Functions/Binary Logic  syn_binlog_exp=a^b  synBlockType=primitive  synLatency=0  synBlockId=13
  Binary Logic2 : shlslibv1/Math Functions/Binary Logic  syn_binlog_exp=a^b  synBlockType=primitive  synLatency=0  synBlockId=13
  Display5 : Display
      settings: Format=hex (Stored Integer)
  Port Out : shlslibv1/Ports & Subsystems/Port Out  syn_capture=on  syn_register=on  synBlockType=port  synLatency=1  synBlockId=1
  multiplier1 : shlslibv1/Memories/ROM  syn_rom_vec=mul11  syn_rom_auto_wl=on  syn_out_wl=8  syn_out_fl=0  syn_out_dt=unsigned  syn_out_sat=on  syn_out_rnd=on  syn_en_port=off  synBlockType=primitive  synLatency=1  synBlockId=62  syn_dual_port=off
  multiplier2 : shlslibv1/Memories/ROM  syn_rom_vec=mul9  syn_rom_auto_wl=on  syn_out_wl=8  syn_out_fl=0  syn_out_dt=unsigned  syn_out_sat=on  syn_out_rnd=on  syn_en_port=off  synBlockType=primitive  synLatency=1  synBlockId=62  syn_dual_port=off
  multiplier3 : shlslibv1/Memories/ROM  syn_rom_vec=mul14  syn_rom_auto_wl=on  syn_out_wl=8  syn_out_fl=0  syn_out_dt=unsigned  syn_out_sat=on  syn_out_rnd=on  syn_en_port=off  synBlockType=primitive  synLatency=1  synBlockId=62  syn_dual_port=off
  multiplier4 : shlslibv1/Memories/ROM  syn_rom_vec=mul13  syn_rom_auto_wl=on  syn_out_wl=8  syn_out_fl=0  syn_out_dt=unsigned  syn_out_sat=on  syn_out_rnd=on  syn_en_port=off  synBlockType=primitive  synLatency=1  synBlockId=62  syn_dual_port=off
  Out1 : Outport
  wires:
  multiplier3/1 -> Binary Logic/2
  In2/1 -> multiplier3/1
  multiplier2/1 -> Binary Logic/1
  Binary Logic2/1 -> Port Out/1, Out1/1
  In1/1 -> multiplier2/1
  Port Out/1 -> Display5/1
  Binary Logic/1 -> Binary Logic2/1
  Binary Logic1/1 -> Binary Logic2/2
  multiplier1/1 -> Binary Logic1/1
  In3/1 -> multiplier1/1
  multiplier4/1 -> Binary Logic1/2
  In4/1 -> multiplier4/1

== system aes_impl_decrypt_smc/Round14/Subsystem8/Subsystem6/Mixcolumn2 ==
  In1 : Inport
  In2 : Inport  Port=2
  In3 : Inport  Port=3
  In4 : Inport  Port=4
  Binary Logic : shlslibv1/Math Functions/Binary Logic  syn_binlog_exp=a^b  synBlockType=primitive  synLatency=0  synBlockId=13
  Binary Logic1 : shlslibv1/Math Functions/Binary Logic  syn_binlog_exp=a^b  synBlockType=primitive  synLatency=0  synBlockId=13
  Binary Logic2 : shlslibv1/Math Functions/Binary Logic  syn_binlog_exp=a^b  synBlockType=primitive  synLatency=0  synBlockId=13
  Display5 : Display
      settings: Format=hex (Stored Integer)
  Port Out : shlslibv1/Ports & Subsystems/Port Out  syn_capture=on  syn_register=on  synBlockType=port  synLatency=1  synBlockId=1
  multiplier1 : shlslibv1/Memories/ROM  syn_rom_vec=mul14  syn_rom_auto_wl=on  syn_out_wl=8  syn_out_fl=0  syn_out_dt=unsigned  syn_out_sat=on  syn_out_rnd=on  syn_en_port=off  synBlockType=primitive  synLatency=1  synBlockId=62  syn_dual_port=off
  multiplier2 : shlslibv1/Memories/ROM  syn_rom_vec=mul13  syn_rom_auto_wl=on  syn_out_wl=8  syn_out_fl=0  syn_out_dt=unsigned  syn_out_sat=on  syn_out_rnd=on  syn_en_port=off  synBlockType=primitive  synLatency=1  synBlockId=62  syn_dual_port=off
  multiplier3 : shlslibv1/Memories/ROM  syn_rom_vec=mul9  syn_rom_auto_wl=on  syn_out_wl=8  syn_out_fl=0  syn_out_dt=unsigned  syn_out_sat=on  syn_out_rnd=on  syn_en_port=off  synBlockType=primitive  synLatency=1  synBlockId=62  syn_dual_port=off
  multiplier4 : shlslibv1/Memories/ROM  syn_rom_vec=mul11  syn_rom_auto_wl=on  syn_out_wl=8  syn_out_fl=0  syn_out_dt=unsigned  syn_out_sat=on  syn_out_rnd=on  syn_en_port=off  synBlockType=primitive  synLatency=1  synBlockId=62  syn_dual_port=off
  Out1 : Outport
  wires:
  multiplier3/1 -> Binary Logic/2
  In2/1 -> multiplier3/1
  multiplier2/1 -> Binary Logic/1
  Binary Logic2/1 -> Port Out/1, Out1/1
  In1/1 -> multiplier2/1
  Port Out/1 -> Display5/1
  Binary Logic/1 -> Binary Logic2/1
  Binary Logic1/1 -> Binary Logic2/2
  multiplier1/1 -> Binary Logic1/1
  In3/1 -> multiplier1/1
  multiplier4/1 -> Binary Logic1/2
  In4/1 -> multiplier4/1

== system aes_impl_decrypt_smc/Round14/Subsystem8/Subsystem6/Mixcolumn3 ==
  In1 : Inport
  In2 : Inport  Port=2
  In3 : Inport  Port=3
  In4 : Inport  Port=4
  Binary Logic : shlslibv1/Math Functions/Binary Logic  syn_binlog_exp=a^b  synBlockType=primitive  synLatency=0  synBlockId=13
  Binary Logic1 : shlslibv1/Math Functions/Binary Logic  syn_binlog_exp=a^b  synBlockType=primitive  synLatency=0  synBlockId=13
  Binary Logic2 : shlslibv1/Math Functions/Binary Logic  syn_binlog_exp=a^b  synBlockType=primitive  synLatency=0  synBlockId=13
  Display5 : Display
      settings: Format=hex (Stored Integer)
  Port Out : shlslibv1/Ports & Subsystems/Port Out  syn_capture=on  syn_register=on  synBlockType=port  synLatency=1  synBlockId=1
  multiplier1 : shlslibv1/Memories/ROM  syn_rom_vec=mul9  syn_rom_auto_wl=on  syn_out_wl=8  syn_out_fl=0  syn_out_dt=unsigned  syn_out_sat=on  syn_out_rnd=on  syn_en_port=off  synBlockType=primitive  synLatency=1  synBlockId=62  syn_dual_port=off
  multiplier2 : shlslibv1/Memories/ROM  syn_rom_vec=mul11  syn_rom_auto_wl=on  syn_out_wl=8  syn_out_fl=0  syn_out_dt=unsigned  syn_out_sat=on  syn_out_rnd=on  syn_en_port=off  synBlockType=primitive  synLatency=1  synBlockId=62  syn_dual_port=off
  multiplier3 : shlslibv1/Memories/ROM  syn_rom_vec=mul13  syn_rom_auto_wl=on  syn_out_wl=8  syn_out_fl=0  syn_out_dt=unsigned  syn_out_sat=on  syn_out_rnd=on  syn_en_port=off  synBlockType=primitive  synLatency=1  synBlockId=62  syn_dual_port=off
  multiplier4 : shlslibv1/Memories/ROM  syn_rom_vec=mul14  syn_rom_auto_wl=on  syn_out_wl=8  syn_out_fl=0  syn_out_dt=unsigned  syn_out_sat=on  syn_out_rnd=on  syn_en_port=off  synBlockType=primitive  synLatency=1  synBlockId=62  syn_dual_port=off
  Out1 : Outport
  wires:
  multiplier3/1 -> Binary Logic/2
  In2/1 -> multiplier3/1
  multiplier2/1 -> Binary Logic/1
  Binary Logic2/1 -> Port Out/1, Out1/1
  In1/1 -> multiplier2/1
  Port Out/1 -> Display5/1
  Binary Logic/1 -> Binary Logic2/1
  Binary Logic1/1 -> Binary Logic2/2
  multiplier1/1 -> Binary Logic1/1
  In3/1 -> multiplier1/1
  multiplier4/1 -> Binary Logic1/2
  In4/1 -> multiplier4/1
